simulink model "text005"  (R2020b)
settings: Solver=VariableStepAuto  StartTime=0.0  StopTime=10.0  RelTol=1e-3
libraries: powerlib x13, eeDiscretePi x1, powerlib_extras x1
settings Model: Creator=38061  LastModifiedBy=38061

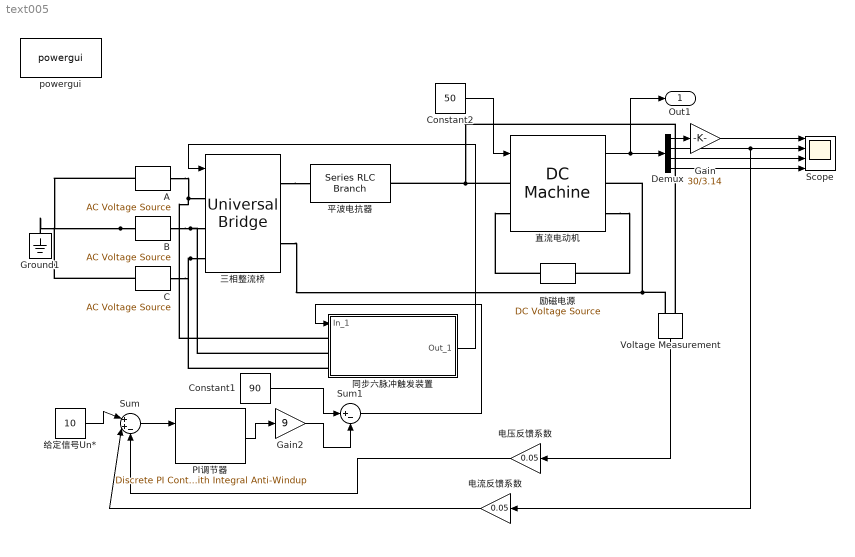
== system text005 ==
  A : powerlib/Electrical Sources/AC Voltage Source  Amplitude=220  Phase=0  Frequency=50  SampleTime=0  Measurements=None  BusType=swing  Pref=10e3  Qref=0  Qmin=-inf  Qmax=+inf
  B : powerlib/Electrical Sources/AC Voltage Source  Amplitude=220  Phase=120  Frequency=50  SampleTime=0  Measurements=None  BusType=swing  Pref=10e3  Qref=0  Qmin=-inf  Qmax=+inf
  C : powerlib/Electrical Sources/AC Voltage Source  Amplitude=220  Phase=240  Frequency=50  SampleTime=0  Measurements=None  BusType=swing  Pref=10e3  Qref=0  Qmin=-inf  Qmax=+inf
  Constant1 : Constant  Value=90
  Constant2 : Constant  Value=50
  Demux : Demux
  Gain : Gain  Gain=30/3.14
  Gain2 : Gain  Gain=9
  Ground1 : powerlib/Elements/Ground  LConnTagsString=a
  PI调节器 : eeDiscretePi/Discrete PI Controller with Integral Anti-Windup  Kp=0.1  Ki=1  x0=0  B=10  A=-10  Ts=50e-6
      settings: SourceProductBaseCode=PS
  Scope : Scope  NumInputPorts=4
  Sum : Sum  Inputs=|++-
  Sum1 : Sum  Inputs=|+-
  Voltage Measurement : powerlib/Measurements/Voltage Measurement  PhasorSimulation=off  OutputType=Complex  PSBequivalent=0
  powergui : powerlib/powergui  Priority=1  SimulationMode=Continuous  SampleTime=50e-6  frequency=60  Iterations=50  frequencyindice=50  Pbase=100e6  ErrMax=1e-4  UnitsV=kV  UnitsW=MW  buscounter=0  FunctionMessages=off  echomessages=off  EnableUseOfTLC=off  CurrentSourceSwitches=off  DisableSnubberDevices=off  DisableRonSwitches=off  DisableVfSwitches=off  DisplayEquations=off  AutomaticDiscreteSolvers=off  SolverType=Tustin/Backward Euler (TBE)  Interpol=off  ExternalGateDelay=off  methode=off  Ts=100  x0status=blocks  SPID=on  SwTol=0  HookPort=off  NonlinearTolerance=1e-4  nMaxIteration=100  ContinueOnMaxIteration=off  RestoreLinks=warning  ResistiveCurrentMeasurement=off  Frange=[0:2:500]  Ylog=off  Xlog=on  ShowGrid=off  save=off  variable=ZData  structure=0  ZoomFFT=off  StartTime=0.0  cycles=1  DisplayStyle=1  fundamental=60  FreqAxis=off  MaxFrequency=1000  frequencyindicesteady=1  RmsSteady=1  display=off
  三相整流桥 : powerlib/Power Electronics/Universal Bridge  Arms=3  SnubberResistance=1e5  SnubberCapacitance=inf  Device=Thyristors  Ron=1e-3  Lon=0  ForwardVoltages="[  0  0  ]"  ForwardVoltage=0  GTOparameters=[ 10e-6 , 20e-6 ]  IGBTparameters=[ 1e-6 , 2e-6 ]  Measurements=None  Measurements_2=None  converterType=Rectifier
  励磁电源 : powerlib/Electrical Sources/DC Voltage Source  Amplitude=220  Measurements=None
  同步六脉冲触发装置 : Subsystem
  平波电抗器 : powerlib/Elements/Series RLC Branch  LConnTagsString=__new0  RConnTagsString=__new0  BranchType=L  Resistance=0  Inductance=1e-3  SetiL0=off  InitialCurrent=0  Capacitance=inf  Setx0=off  InitialVoltage=0  Measurements=None
  电压反馈系数 : Gain  Gain=0.05
  电流反馈系数 : Gain  Gain=0.05
  直流电动机 : powerlib/Machines/DC Machine  PresetModel=No  MechanicalLoad=Torque TL  FieldType=Wound  ShowDetailedParameters=on  MeasurementBus=off  RLa="[ 0.6  0.012]"  RLf="[ 240  120]"  Laf=1.8  MachineConstant=Torque constant (N.m/A)  Ke=1.8  Kt=1.8  J=1  Bm=0  Tf=0  w0=1  Ifinit=0.916666666666667  TsPowergui=0  TsBlock=-1
  给定信号Un* : Constant  Value=10
  Out1 : Outport
  wires:
  Sum1/1 -> 同步六脉冲触发装置/1(In_1)
  直流电动机/1 -> Out1/1, Demux/1
  Demux/3 -> Scope/3
  同步六脉冲触发装置/1(Out_1) -> 三相整流桥/1
  PI调节器/1 -> Gain2/1
  Demux/4 -> Scope/4
  Demux/2 -> 电流反馈系数/1, Scope/2
  Sum/1 -> PI调节器/1
  Constant1/1 -> Sum1/1
  Gain2/1 -> Sum1/2
  给定信号Un*/1 -> Sum/1
  Constant2/1 -> 直流电动机/1
  Gain/1 -> Scope/1
  Demux/1 -> Gain/1
  电流反馈系数/1 -> Sum/2
  Voltage Measurement/1 -> 电压反馈系数/1
  电压反馈系数/1 -> Sum/3
  connections:
  同步六脉冲触发装置/LConn1 -- 三相整流桥/LConn1 -- A/RConn1
  同步六脉冲触发装置/LConn2 -- 三相整流桥/LConn2 -- B/RConn1
  B/LConn1 -- Ground1/LConn1 -- C/LConn1 -- A/LConn1
  三相整流桥/LConn3 -- C/RConn1 -- 同步六脉冲触发装置/LConn3
  直流电动机/RConn2 -- 励磁电源/LConn1
  三相整流桥/RConn2 -- Voltage Measurement/LConn2 -- 直流电动机/RConn1
  直流电动机/LConn1 -- 平波电抗器/RConn1 -- Voltage Measurement/LConn1
  三相整流桥/RConn1 -- 平波电抗器/LConn1
  励磁电源/RConn1 -- 直流电动机/LConn2

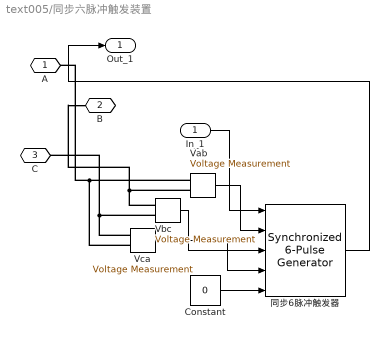
== system text005/同步六脉冲触发装置 ==
  In_1 : Inport
  Constant : Constant  Value=0
  Vab : powerlib/Measurements/Voltage Measurement  PhasorSimulation=off  OutputType=Complex  PSBequivalent=0
  Vbc : powerlib/Measurements/Voltage Measurement  PhasorSimulation=off  OutputType=Complex  PSBequivalent=0
  Vca : powerlib/Measurements/Voltage Measurement  PhasorSimulation=off  OutputType=Complex  PSBequivalent=0
  同步6脉冲触发器 : powerlib_extras/Control  Blocks/Synchronized 6-Pulse Generator  freq=50  pwidth=10  Double_Pulse=off
      settings: SourceProductBaseCode=PS
  A : PMIOPort  Side=Left
  B : PMIOPort  Port=2  Side=Left
  C : PMIOPort  Port=3  Side=Left
  Out_1 : Outport
  wires:
  同步6脉冲触发器/1 -> Out_1/1
  Vca/1 -> 同步6脉冲触发器/4
  Vab/1 -> 同步6脉冲触发器/2
  Constant/1 -> 同步6脉冲触发器/5
  Vbc/1 -> 同步6脉冲触发器/3
  In_1/1 -> 同步6脉冲触发器/1
  connections:
  Vca/LConn1 -- Vbc/LConn2 -- C/RConn1
  Vca/LConn2 -- Vab/LConn1 -- A/RConn1
  Vbc/LConn1 -- Vab/LConn2 -- B/RConn1
